simulink model "Motor"  (R2017a)
settings: Solver=ode45  StartTime=0.0  StopTime=1  RelTol=1e-3
values from neighbouring files (symbols this model uses):
  b = 1.1    [Continuo.m]    (also in Discreto.m)
  ici = 10    [Continuo.m]
  J = 15    [Continuo.m]    (also in Discreto.m)
  K = 6.69    [Continuo.m]    (also in Discreto.m)
  L = 0.00279    [Continuo.m]    (also in Discreto.m)
  R = 0.051    [Continuo.m]    (also in Discreto.m)
  T = 0    [Continuo.m]
  U = [real(V1),imag(V1)]    [Continuo.m]    (also in Planos.m)
  wci = 65    [Continuo.m]
settings Model: Creator=joaqu  LastModifiedBy=joaqu
settings DataIOCC: LimitDataPoints=on  SaveFormat=Array  Refine=10
settings OptimizationCC: BlockReduction=off  BooleanDataType=off  LifeSpan=inf
settings DebuggingCC: SaveWithParameterizedLinksMsg=none  UnderspecifiedInitializationDetection=Classic  MergeDetectMultiDrivingBlocksExec=none  SignalResolutionControl=TryResolveAllWithWarning  SFUnexpectedBacktrackingDiag=warning  SFNoUnconditionalDefaultTransitionDiag=warning  SFExecutionAtInitializationDiag=none
settings HardwareCC: ProdBitPerPointer=32  ProdBitPerSizeT=32  ProdBitPerPtrDiffT=32  ProdLargestAtomicFloat=None  ProdIntDivRoundTo=Undefined  ProdEndianess=Unspecified  ProdWordSize=32  ProdHWDeviceType=32-bit Generic  TargetUnknown=on
settings ModelReferenceCC: PropagateSignalLabelsOutOfModel=off
settings GRTTargetCC: TargetLangStandard=C89/C90 (ANSI)  GeneratePreprocessorConditionals=Disable all
settings ConfigComp: CovMetricSettings=dw  CovHtmlReporting=on  CovSaveCumulativeToWorkspaceVar=on  CovSaveSingleToWorkspaceVar=on  CovExternalEMLEnable=off  CovSFcnEnable=off

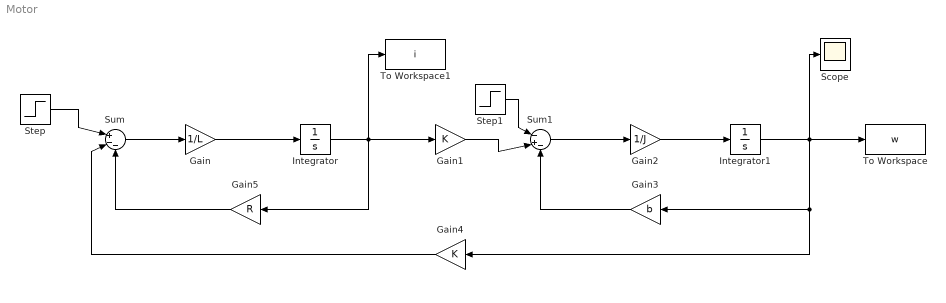
== system Motor ==
  Gain : Gain  Gain=1/L
  Gain1 : Gain  Gain=K
  Gain2 : Gain  Gain=1/J
  Gain3 : Gain  Gain=b
  Gain4 : Gain  Gain=K
  Gain5 : Gain  Gain=R
  Integrator : Integrator  InitialCondition=ici
  Integrator1 : Integrator  InitialCondition=wci
  Scope : Scope
  Step : Step  Time=0  After=U  SampleTime=0
  Step1 : Step  Time=0  After=T  SampleTime=0
  Sum : Sum  Inputs=|+--
  Sum1 : Sum  Inputs=|-+-
  To Workspace : ToWorkspace  VariableName=w  SaveFormat=Timeseries  SampleTime=-1
  To Workspace1 : ToWorkspace  VariableName=i  SaveFormat=Timeseries  SampleTime=-1
  wires:
  Sum/1 -> Gain/1
  Gain/1 -> Integrator/1
  Integrator/1 -> To Workspace1/1, Gain5/1, Gain1/1
  Sum1/1 -> Gain2/1
  Gain2/1 -> Integrator1/1
  Gain5/1 -> Sum/3
  Gain4/1 -> Sum/2
  Integrator1/1 -> Gain4/1, Gain3/1, To Workspace/1, Scope/1
  Gain1/1 -> Sum1/2
  Gain3/1 -> Sum1/3
  Step/1 -> Sum/1
  Step1/1 -> Sum1/1
